simulink model "Vaccum_circuit_w_load_forward"  (R2022a)
settings: Solver=FixedStepAuto  StartTime=0.0  StopTime=.004  FixedStep=SampleTime  RelTol=1e-3
values from neighbouring files (symbols this model uses):
  Ad = sys_d_plasma.A    [All_injectors_LQG_bop_plasma_ss_model_code.m]    (also in All_injectors_LQG_bop_ss_model_code.m; All_injectors_LQG_continuous_time_code.m; All_injectors_LQG_plasma_7_15_24_code.m; All_injectors_LQG_plasma_ss_model_code.m)
  Amplitude = 600    [All_injectors_LQG_bop_plasma_ss_model_code.m]    (also in All_injectors_LQG_bop_ss_model_code.m; All_injectors_LQG_continuous_time_code.m; All_injectors_LQG_plasma_7_15_24_code.m; All_injectors_LQG_plasma_ss_model_code.m)
  Bd = sys_d_plasma.B    [All_injectors_LQG_bop_plasma_ss_model_code.m]    (also in All_injectors_LQG_bop_ss_model_code.m; All_injectors_LQG_continuous_time_code.m; All_injectors_LQG_plasma_7_15_24_code.m; All_injectors_LQG_plasma_ss_model_code.m)
  Cap = 96e-6    (= 9.6e-05)    [All_injectors_LQG_bop_ss_model_code.m]    (also in All_injectors_LQG_continuous_time_code.m; All_injectors_LQG_plasma_7_15_24_code.m; All_injectors_LQG_plasma_ss_model_code.m; All_injectors_vaccum.m)
  Cd = sys_d_plasma.C    [All_injectors_LQG_bop_plasma_ss_model_code.m]    (also in All_injectors_LQG_bop_ss_model_code.m; All_injectors_LQG_continuous_time_code.m; All_injectors_LQG_plasma_7_15_24_code.m; All_injectors_LQG_plasma_ss_model_code.m)
  Dd = sys_d_plasma.D    [All_injectors_LQG_bop_plasma_ss_model_code.m]    (also in All_injectors_LQG_bop_ss_model_code.m; All_injectors_LQG_continuous_time_code.m; All_injectors_LQG_plasma_7_15_24_code.m; All_injectors_LQG_plasma_ss_model_code.m)
  L1 = (9.78e-7)    (= 9.78e-07)    [All_injectors_LQG_bop_plasma_ss_model_code.m]    (also in All_injectors_LQG_bop_ss_model_code.m = 8.0141e-07; All_injectors_LQG_continuous_time_code.m = 8.0141e-07; All_injectors_LQG_plasma_7_15_24_code.m = 8.0141e-07; All_injectors_LQG_plasma_ss_model_code.m = 8.0141e-07)
  L2 = 2.0462e-6    (= 2.0462e-06)    [All_injectors_LQG_bop_ss_model_code.m]    (also in All_injectors_LQG_continuous_time_code.m; All_injectors_LQG_plasma_7_15_24_code.m; All_injectors_LQG_plasma_ss_model_code.m; All_injectors_vaccum.m)
  Lp = L2    (= 2.0462e-06)    [All_injectors_LQG_bop_ss_model_code.m]    (also in All_injectors_LQG_continuous_time_code.m; All_injectors_LQG_plasma_7_15_24_code.m; All_injectors_LQG_plasma_ss_model_code.m; Plasma_ss_model.m = 1.0231e-06)
  R = 1    [All_injectors_LQG_bop_plasma_ss_model_code.m]    (also in All_injectors_LQG_bop_ss_model_code.m = diag(1*ones(1,num_inputs)); All_injectors_LQG_continuous_time_code.m = diag(1*ones(1,num_inputs)); All_injectors_LQG_plasma_7_15_24_code.m = diag(1*ones(1,num_inputs)); All_injectors_LQG_plasma_ss_model_code.m = diag(1*ones(1,num_inputs)))
  R1 = .0025    (= 0.0025)    [All_injectors_LQG_bop_ss_model_code.m]    (also in All_injectors_LQG_continuous_time_code.m; All_injectors_LQG_plasma_7_15_24_code.m; All_injectors_LQG_plasma_ss_model_code.m; All_injectors_vaccum.m)
  R2 = .005    (= 0.005)    [All_injectors_LQG_bop_ss_model_code.m]    (also in All_injectors_LQG_continuous_time_code.m; All_injectors_LQG_plasma_7_15_24_code.m; All_injectors_LQG_plasma_ss_model_code.m; All_injectors_vaccum.m)
  R3 = .005    (= 0.005)    [All_injectors_LQG_bop_ss_model_code.m]    (also in All_injectors_LQG_continuous_time_code.m; All_injectors_LQG_plasma_7_15_24_code.m; All_injectors_LQG_plasma_ss_model_code.m; All_injectors_vaccum.m)
  RunTime = .004    (= 0.004)    [All_injectors_LQG_bop_plasma_ss_model_code.m]    (also in All_injectors_LQG_bop_ss_model_code.m; All_injectors_LQG_continuous_time_code.m; All_injectors_LQG_plasma_7_15_24_code.m; All_injectors_LQG_plasma_ss_model_code.m)
  SampleTime = 1e-7    (= 1e-07)    [All_injectors_LQG_bop_plasma_ss_model_code.m]    (also in All_injectors_LQG_bop_ss_model_code.m; All_injectors_LQG_continuous_time_code.m; All_injectors_LQG_plasma_7_15_24_code.m; All_injectors_LQG_plasma_ss_model_code.m)
  voltage = Amplitude*sin(2*pi*Frequency*time)    [All_injectors_LQG_bop_plasma_ss_model_code.m]    (also in All_injectors_LQG_bop_ss_model_code.m; All_injectors_LQG_continuous_time_code.m; All_injectors_LQG_plasma_7_15_24_code.m; All_injectors_LQG_plasma_ss_model_code.m)
undefined symbols (not defined in the file or in its folder): Discrete, Time
libraries: spsSeriesRLCBranchLib x10, spsMosfetLib x4, spsVoltageMeasurementLib x4, simulink x4, spsDCVoltageSourceLib x3, spsCurrentMeasurementLib x3, spsFullBridgeMMCExternalDCLinksLib x2, spsPWMGeneratorMultilevelLib x2, ctrlSharedLib x1, spspowerguiLib x1
settings Model: Creator=ducks  LastModifiedBy=ducks
settings DataIOCC: ExternalInput=[t,V]

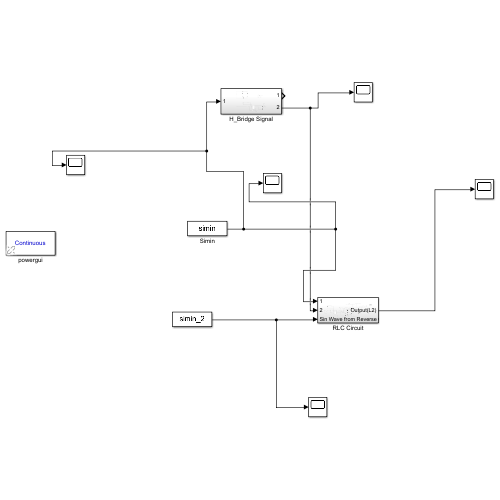
[thumbnail: Simulink's stored preview of the top-level diagram]
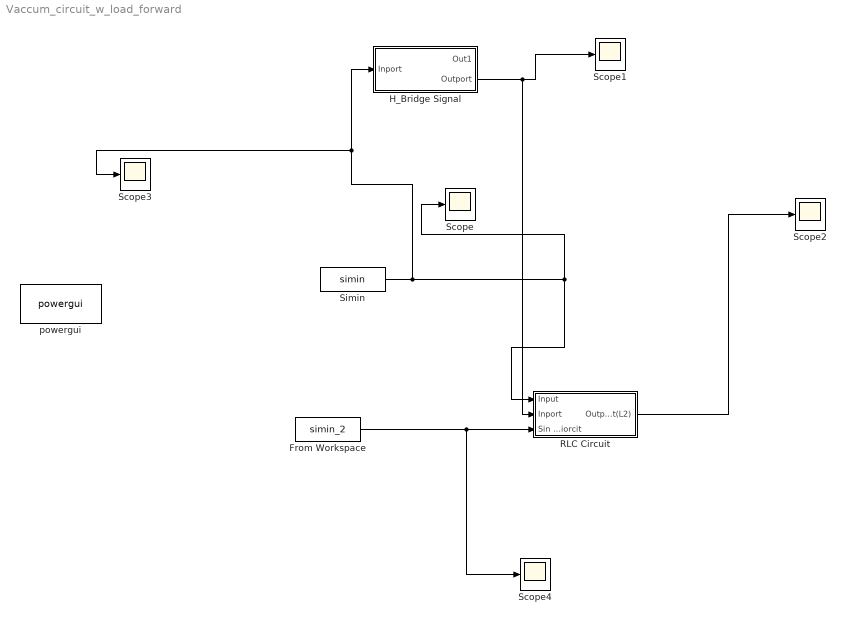
== system Vaccum_circuit_w_load_forward ==
  From Workspace : FromWorkspace  VariableName=simin_2
  H_Bridge Signal : Subsystem
  RLC Circuit : Subsystem
  Scope{,1..4} (5 alike) : Scope
  Simin : FromWorkspace  VariableName=simin
  powergui : spspowerguiLib/powergui  Priority=1  SimulationMode=Continuous  SampleTime=50e-6  frequency=60  Iterations=50  frequencyindice=0  Pbase=100e6  ErrMax=1e-4  UnitsV=kV  UnitsW=MW  buscounter=0  FunctionMessages=off  echomessages=off  EnableUseOfTLC=off  CurrentSourceSwitches=off  DisableSnubberDevices=off  DisableRonSwitches=off  DisableVfSwitches=off  DisplayEquations=off  AutomaticDiscreteSolvers=off  SolverType=Tustin/Backward Euler (TBE)  Interpol=off  ExternalGateDelay=off  methode=off  Ts=100  x0status=blocks  SPID=on  SwTol=0  HookPort=off  NonlinearTolerance=1e-4  nMaxIteration=100  ContinueOnMaxIteration=off  RestoreLinks=warning  ResistiveCurrentMeasurement=off  Frange=[0:2:500]  Ylog=off  Xlog=on  ShowGrid=off  save=off  variable=ZData  structure=0  ZoomFFT=off  StartTime=0.0  cycles=1  DisplayStyle=1  fundamental=60  FreqAxis=off  MaxFrequency=1000  frequencyindicesteady=1  RmsSteady=1  display=off
  wires:
  Simin/1 -> Scope3/1, H_Bridge Signal/1(Inport), Scope/1, RLC Circuit/1(Input)
  RLC Circuit/1(Output(L2)) -> Scope2/1
  H_Bridge Signal/2(Outport) -> RLC Circuit/2(Inport), Scope1/1
  From Workspace/1 -> Scope4/1, RLC Circuit/3(Sin Wave from Reverse Ciorcit)

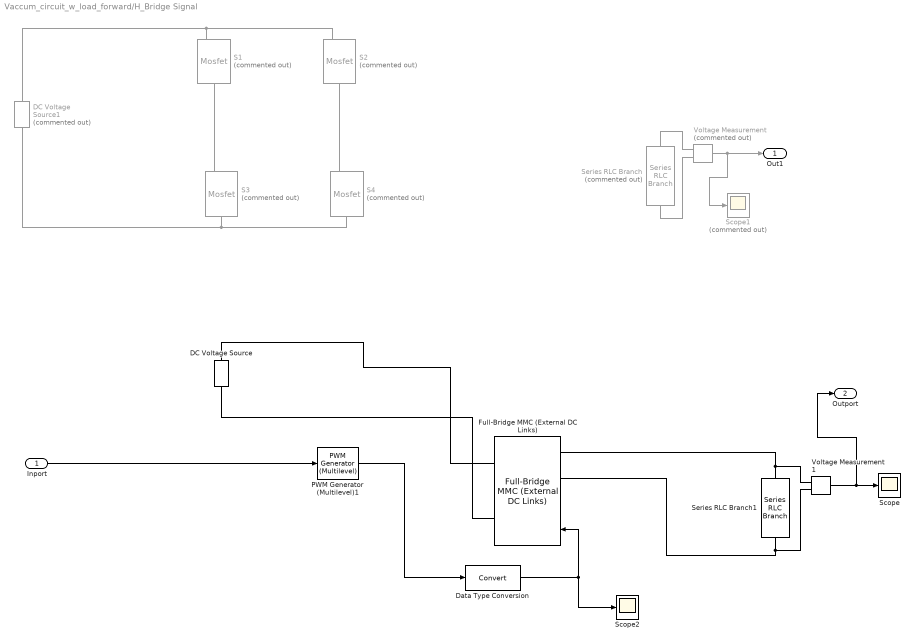
== system Vaccum_circuit_w_load_forward/H_Bridge Signal ==
  Inport : Inport
  DC Voltage Source : spsDCVoltageSourceLib/DC Voltage Source  Amplitude=600  Measurements=None
  DC Voltage Source1 : spsDCVoltageSourceLib/DC Voltage Source  Commented=on  Amplitude=600  Measurements=None
  Data Type Conversion : DataTypeConversion  SaturateOnIntegerOverflow=off  RndMeth=Floor
  Full-Bridge MMC (External DC Links) : spsFullBridgeMMCExternalDCLinksLib/Full-Bridge MMC (External DC Links)  ModelType=Switching devices  n=1  Ron=1e-3  Rs=1e6  Cs=inf  Ron_Diode=1e-3  Rs_Diode=1e6  Cs_Diode=inf  Vf_Diode=1e-3  Rs_CurrentSource=inf  Ts=10e-6
      settings: SourceProductBaseCode=PS
  PWM Generator (Multilevel)1 : spsPWMGeneratorMultilevelLib/PWM Generator (Multilevel)  BridgeType=Full-bridge  NumberOfBridges=1  Fc=1e3  Ts=0  ShowCarriersOutport=off
      settings: SourceProductBaseCode=PS
  S{1..4} (4 alike) : spsMosfetLib/Mosfet  Commented=on  Ron=0.1  Lon=0  Rd=0.01  Vfd=0  IC=0  Rs=1e5  Cs=inf  Measurements=off
  Scope : Scope
  Scope1 : Scope  Commented=on
  Scope2 : Scope
  Series RLC Branch : spsSeriesRLCBranchLib/Series RLC Branch  Commented=on  LConnTagsString=__new0  RConnTagsString=__new0  BranchType=R  Resistance=1  Inductance=1e-3  SetiL0=off  InitialCurrent=0  Capacitance=1e-6  Setx0=off  InitialVoltage=0  Measurements=None
  Series RLC Branch1 : spsSeriesRLCBranchLib/Series RLC Branch  LConnTagsString=__new0  RConnTagsString=__new0  BranchType=R  Resistance=1  Inductance=1e-3  SetiL0=off  InitialCurrent=0  Capacitance=1e-6  Setx0=off  InitialVoltage=0  Measurements=None
  Voltage Measurement : spsVoltageMeasurementLib/Voltage Measurement  Commented=on  PhasorSimulation=off  OutputType=Complex  PSBequivalent=0
  Voltage Measurement1 : spsVoltageMeasurementLib/Voltage Measurement  PhasorSimulation=off  OutputType=Complex  PSBequivalent=0
  Out1 : Outport
  Outport : Outport  Port=2
  wires:
  Voltage Measurement/1 -> Scope1/1, Out1/1
  PWM Generator (Multilevel)1/1 -> Data Type Conversion/1
  Inport/1 -> PWM Generator (Multilevel)1/1
  Data Type Conversion/1 -> Full-Bridge MMC (External DC Links)/1, Scope2/1
  Voltage Measurement1/1 -> Outport/1, Scope/1
  connections:
  Voltage Measurement/LConn1 -- Series RLC Branch/LConn1
  Voltage Measurement/LConn2 -- Series RLC Branch/RConn1
  S1/LConn1 -- S2/LConn1 -- DC Voltage Source1/LConn1
  S1/RConn1 -- S3/LConn1
  S3/RConn1 -- DC Voltage Source1/RConn1 -- S4/RConn1
  S4/LConn1 -- S2/RConn1
  Full-Bridge MMC (External DC Links)/LConn1 -- Voltage Measurement1/LConn2 -- Series RLC Branch1/RConn1
  Full-Bridge MMC (External DC Links)/RConn2 -- DC Voltage Source/LConn1
  Full-Bridge MMC (External DC Links)/LConn2 -- Voltage Measurement1/LConn1 -- Series RLC Branch1/LConn1
  Full-Bridge MMC (External DC Links)/RConn1 -- DC Voltage Source/RConn1

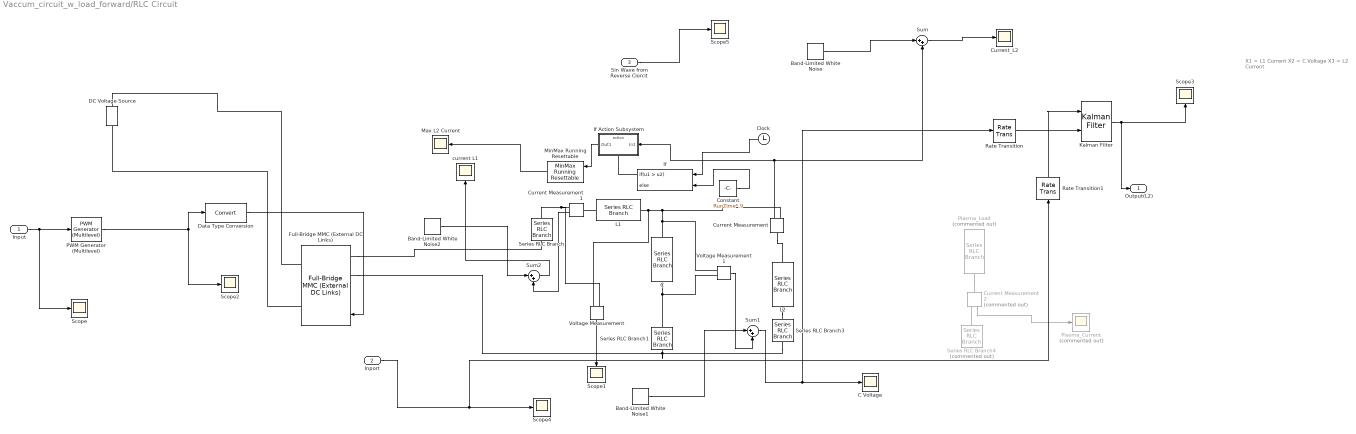
== system Vaccum_circuit_w_load_forward/RLC Circuit ==
  note: X1 = L1 Current
      | X2 = C Voltage
      | X3 = L2 Current
  Input : Inport
  Inport : Inport  Port=2
  Sin Wave from Reverse Ciorcit : Inport  Port=3
  Band-Limited White Noise : simulink/Sources/Band-Limited White Noise  Cov=NoisePower  Ts=SampleTime  seed=[23341]
  Band-Limited White Noise1 : simulink/Sources/Band-Limited White Noise  Cov=NoisePower  Ts=SampleTime  seed=[23341]
  Band-Limited White Noise2 : simulink/Sources/Band-Limited White Noise  Cov=NoisePower  Ts=SampleTime  seed=[23341]
  C : spsSeriesRLCBranchLib/Series RLC Branch  LConnTagsString=__new0  RConnTagsString=__new0  BranchType=C  Resistance=1  Inductance=1e-3  SetiL0=off  InitialCurrent=0  Capacitance=Cap  Setx0=off  InitialVoltage=0  Measurements=None
  C Voltage : Scope
  Clock : Clock
  Constant : Constant  Value=RunTime*.9
  Current Measurement : spsCurrentMeasurementLib/Current Measurement  PhasorSimulation=off  OutputType=Complex  PSBequivalent=0
  Current Measurement1 : spsCurrentMeasurementLib/Current Measurement  PhasorSimulation=off  OutputType=Complex  PSBequivalent=0
  Current Measurement2 : spsCurrentMeasurementLib/Current Measurement  Commented=on  PhasorSimulation=off  OutputType=Complex  PSBequivalent=0
  Current_L2 : Scope
  DC Voltage Source : spsDCVoltageSourceLib/DC Voltage Source  Amplitude=Amplitude  Measurements=None
  Data Type Conversion : DataTypeConversion  SaturateOnIntegerOverflow=off  RndMeth=Floor
  Full-Bridge MMC (External DC Links) : spsFullBridgeMMCExternalDCLinksLib/Full-Bridge MMC (External DC Links)  ModelType=Switching devices  n=1  Ron=1e-3  Rs=1e6  Cs=inf  Ron_Diode=1e-3  Rs_Diode=1e6  Cs_Diode=inf  Vf_Diode=1e-3  Rs_CurrentSource=inf  Ts=1e-6
      settings: SourceProductBaseCode=PS
  If : If  NumInputs=2  IfExpression=u1 > u2
  If Action Subsystem : Subsystem  TreatAsAtomicUnit=on
  Kalman Filter : ctrlSharedLib/Kalman Filter  TimeDomain=Discrete-Time  UseCurrentEstimator=on  ModelSource=Individual A, B, C, D matrices  ModelSourceVariable=ss(0.95,1,1,0,1)  A=Ad  B=Bd  C=Cd  D=Dd  NumberOfStates=1  NumberOfInputs=1  NumberOfOutputs=1  InitialEstimateSource=Dialog  X0=voltage(1)  P0=10  UseK=off  UseGH=off  NumberOfProcessNoiseInputs=1  G=G  TimeInvariantG=on  H=0  TimeInvariantH=on  Q=Q  TimeInvariantQ=on  R=R  TimeInvariantR=on  N=0  TimeInvariantN=on  AddInputPort=on  AddEnablePort=off  OutputEstimatedY=off  OutputP=off  Ts=SampleTime
  L1 : spsSeriesRLCBranchLib/Series RLC Branch  LConnTagsString=__new0  RConnTagsString=__new0  BranchType=L  Resistance=1  Inductance=L1  SetiL0=off  InitialCurrent=0  Capacitance=0  Setx0=off  InitialVoltage=0  Measurements=None
  L2 : spsSeriesRLCBranchLib/Series RLC Branch  LConnTagsString=__new0  RConnTagsString=__new0  BranchType=L  Resistance=1  Inductance=L2  SetiL0=off  InitialCurrent=0  Capacitance=1e-6  Setx0=off  InitialVoltage=0  Measurements=None
  Max L2 Current : Scope
  MinMax Running Resettable : simulink/Math Operations/MinMax Running Resettable  Function=max  vinit=0.0
  PWM Generator (Multilevel) : spsPWMGeneratorMultilevelLib/PWM Generator (Multilevel)  BridgeType=Full-bridge  NumberOfBridges=1  Fc=1e3  Ts=0  ShowCarriersOutport=off
      settings: SourceProductBaseCode=PS
  Plasma_Current : Scope  Commented=on
  Plasma_Load : spsSeriesRLCBranchLib/Series RLC Branch  Commented=on  LConnTagsString=__new0  RConnTagsString=__new0  BranchType=L  Resistance=1  Inductance=Lp  SetiL0=off  InitialCurrent=0  Capacitance=1e-6  Setx0=off  InitialVoltage=0  Measurements=None
  Rate Transition : RateTransition
  Rate Transition1 : RateTransition
  Scope{,1..5} (6 alike) : Scope
  Series RLC Branch : spsSeriesRLCBranchLib/Series RLC Branch  LConnTagsString=__new0  RConnTagsString=__new0  BranchType=R  Resistance=R1  Inductance=1e-3  SetiL0=off  InitialCurrent=0  Capacitance=1e-6  Setx0=off  InitialVoltage=0  Measurements=None
  Series RLC Branch1 : spsSeriesRLCBranchLib/Series RLC Branch  LConnTagsString=__new0  RConnTagsString=__new0  BranchType=R  Resistance=R2  Inductance=1e-3  SetiL0=off  InitialCurrent=0  Capacitance=1e-6  Setx0=off  InitialVoltage=0  Measurements=None
  Series RLC Branch3 : spsSeriesRLCBranchLib/Series RLC Branch  LConnTagsString=__new0  RConnTagsString=__new0  BranchType=R  Resistance=R3  Inductance=1e-3  SetiL0=off  InitialCurrent=0  Capacitance=1e-6  Setx0=off  InitialVoltage=0  Measurements=None
  Series RLC Branch4 : spsSeriesRLCBranchLib/Series RLC Branch  Commented=on  LConnTagsString=__new0  RConnTagsString=__new0  BranchType=R  Resistance=.005  Inductance=1e-3  SetiL0=off  InitialCurrent=0  Capacitance=1e-6  Setx0=off  InitialVoltage=0  Measurements=None
  Sum : Sum  Inputs=|++
  Sum1 : Sum  Inputs=|++
  Sum2 : Sum  Inputs=|++
  Voltage Measurement : spsVoltageMeasurementLib/Voltage Measurement  PhasorSimulation=off  OutputType=Complex  PSBequivalent=0
  Voltage Measurement1 : spsVoltageMeasurementLib/Voltage Measurement  PhasorSimulation=off  OutputType=Complex  PSBequivalent=0
  current L1 : Scope
  Output(L2) : Outport
  wires:
  Voltage Measurement/1 -> Scope1/1
  Current Measurement1/1 -> Sum2/2
  MinMax Running Resettable/1 -> Max L2 Current/1
  Clock/1 -> If/1
  Constant/1 -> If/2
  If/1 -> If Action Subsystem/Action
  If Action Subsystem/1(Out1) -> MinMax Running Resettable/1
  PWM Generator (Multilevel)/1 -> Data Type Conversion/1, Scope2/1
  Input/1 -> Scope/1, PWM Generator (Multilevel)/1
  Current Measurement2/1 -> Plasma_Current/1
  Band-Limited White Noise/1 -> Sum/1
  Current Measurement/1 -> Sum/2, If Action Subsystem/1(In1)
  Data Type Conversion/1 -> Full-Bridge MMC (External DC Links)/1
  Kalman Filter/1 -> Scope3/1, Output(L2)/1
  Sum/1 -> Current_L2/1
  Inport/1 -> Rate Transition1/1, Scope4/1
  Sum2/1 -> current L1/1
  Band-Limited White Noise1/1 -> Sum1/1
  Voltage Measurement1/1 -> Sum1/2
  Band-Limited White Noise2/1 -> Sum2/1
  Sum1/1 -> Rate Transition/1, C Voltage/1
  Sin Wave from Reverse Ciorcit/1 -> Scope5/1
  Rate Transition/1 -> Kalman Filter/2
  Rate Transition1/1 -> Kalman Filter/1
  connections:
  Current Measurement1/RConn1 -- Series RLC Branch/LConn1 -- Voltage Measurement/LConn1
  L1/LConn1 -- Current Measurement1/LConn1
  Full-Bridge MMC (External DC Links)/LConn1 -- Series RLC Branch3/RConn1 -- Series RLC Branch1/RConn1
  Full-Bridge MMC (External DC Links)/RConn1 -- DC Voltage Source/RConn1
  Full-Bridge MMC (External DC Links)/RConn2 -- DC Voltage Source/LConn1
  Full-Bridge MMC (External DC Links)/LConn2 -- Series RLC Branch/RConn1
  Plasma_Load/RConn1 -- Current Measurement2/LConn1
  Series RLC Branch4/LConn1 -- Current Measurement2/RConn1
  L2/RConn1 -- Series RLC Branch3/LConn1
  Current Measurement/LConn1 -- L2/LConn1
  Voltage Measurement/LConn2 -- L1/RConn1 -- Current Measurement/RConn1 -- Voltage Measurement1/LConn1 -- C/LConn1
  Series RLC Branch1/LConn1 -- Voltage Measurement1/LConn2 -- C/RConn1

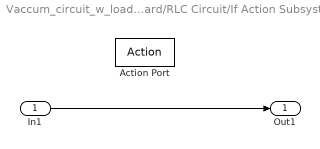
== system Vaccum_circuit_w_load_forward/RLC Circuit/If Action Subsystem ==
  In1 : Inport
  Action Port : ActionPort  ActionPortLabel=if(u1 > u2)
  Out1 : Outport
  wires:
  In1/1 -> Out1/1
